simulink model "Practica6_Simulink"  (R2024a)
settings: Solver=VariableStepAuto  StartTime=0.0  StopTime=0.01  RelTol=1e-6
values from neighbouring files (symbols this model uses):
  C = 10e-6    (= 1e-05)    [DCDC.m]
  L = 2e-3    (= 0.002)    [DCDC.m]
  R = 10    [DCDC.m]
  U = 32    [DCDC.m]
settings Model: Creator=Manuel  LastModifiedBy=Manuel

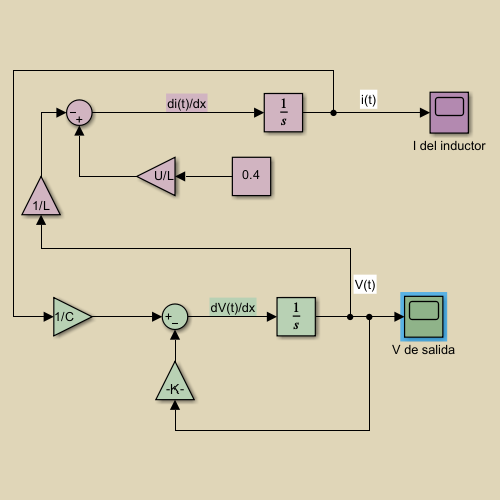
[thumbnail: Simulink's stored preview of the top-level diagram]
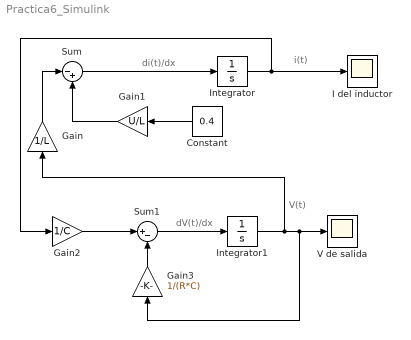
== system Practica6_Simulink ==
  note: di(t)/dx
  note: i(t)
  note: dV(t)/dx
  note: V(t)
  Constant : Constant  Value=0.4
  Gain : Gain  Gain=1/L
  Gain1 : Gain  Gain=U/L
  Gain2 : Gain  Gain=1/C
  Gain3 : Gain  Gain=1/(R*C)
  I del inductor : Scope
  Integrator : Integrator
  Integrator1 : Integrator
  Sum : Sum  Inputs=|-+
  Sum1 : Sum  Inputs=|+-
  V de salida : Scope
  wires:
  Integrator/1 -> I del inductor/1, Gain2/1
  Gain/1 -> Sum/1
  Integrator1/1 -> Gain/1, Gain3/1, V de salida/1
  Constant/1 -> Gain1/1
  Gain1/1 -> Sum/2
  Gain2/1 -> Sum1/1
  Gain3/1 -> Sum1/2
  Sum1/1 -> Integrator1/1
  Sum/1 -> Integrator/1
